simulink model "Model1_Test_Forall"  (R2018b)
settings: Solver=ode8  StartTime=0.0  StopTime=100.0  FixedStep=0.01  RelTol=1e-6
undefined symbols (not defined in the file or in its folder): tollerableriskTest_Forall
settings Model: SimulationMode=accelerator  Creator=claudio.menghi  LastModifiedBy=claudio.menghi
settings SolverCC: MaxConsecutiveZCs=10000  ShapePreserveControl=EnableAll  ZeroCrossControl=EnableAll  ZeroCrossAlgorithm=Adaptive  AutoInsertRateTranBlk=on

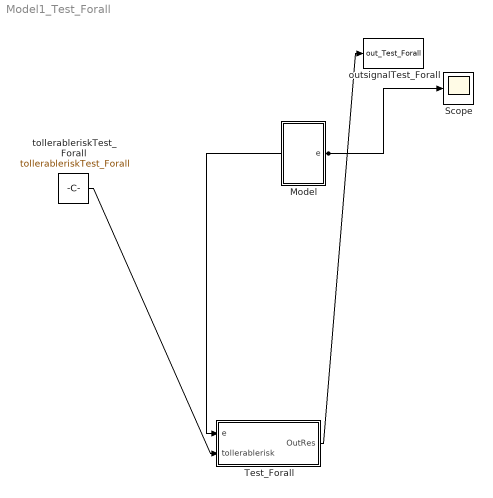
== system Model1_Test_Forall ==
  Model : Subsystem
  Scope : Scope
  Test_Forall : Subsystem
  outsignalTest_Forall : ToWorkspace  VariableName=out_Test_Forall  SaveFormat=Timeseries  SampleTime=-1
      settings: MaxDataPoints=1
  tollerableriskTest_Forall : Constant  Value=tollerableriskTest_Forall
  wires:
  Model/1(e) -> Scope/1, Test_Forall/1(e)
  tollerableriskTest_Forall/1 -> Test_Forall/2(tollerablerisk)
  Test_Forall/1(OutRes) -> outsignalTest_Forall/1

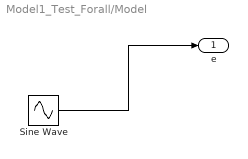
== system Model1_Test_Forall/Model ==
  Sine Wave : Sin  Amplitude=2  SampleTime=0
  e : Outport
  wires:
  Sine Wave/1 -> e/1

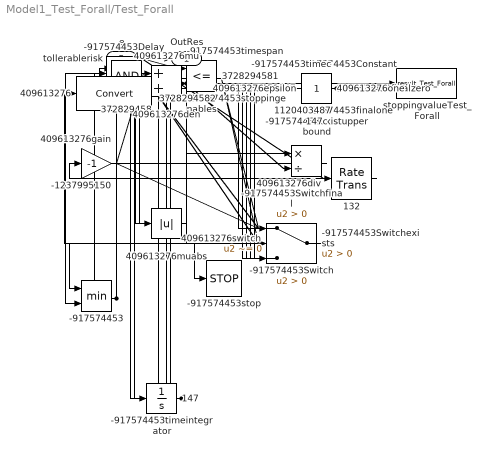
== system Model1_Test_Forall/Test_Forall ==
  e : Inport
  tollerablerisk : Inport  Port=2
  -1237995150 : Gain
  -917574453 : MinMax  Inputs=2
  -917574453Constant : Constant
  -917574453Delay : UnitDelay  InitialCondition=1  SampleTime=-1
  -917574453Switch : Switch  Criteria=u2 > Threshold
  -917574453Switchexists : Switch  Criteria=u2 > Threshold
  -917574453Switchfinal : Switch  Criteria=u2 > Threshold
  -917574453existupperbound : Constant  Value=0.0
  -917574453finalone : Constant
  -917574453finalzero : Constant  Value=0
  -917574453stop : Stop
  -917574453stoppingenables : RelationalOperator  OutDataTypeStr=boolean  RndMeth=Simplest
  -917574453timec : Constant
  -917574453timeintegrator : Integrator
  -917574453timespan : RelationalOperator  OutDataTypeStr=boolean  RndMeth=Simplest
  1065353247 : Constant  Value=1.0
  1120403487 : Constant  Value=100.0
  132 : RateTransition
  147 : Integrator
  147c : Constant
  31 : Constant  Value=0.0
  372829458 : Logic  AllPortsSameDT=off  OutDataTypeStr=boolean
  3728294581 : RelationalOperator  Operator=<=  OutDataTypeStr=boolean  RndMeth=Simplest
  3728294582 : RelationalOperator  Operator=<=  OutDataTypeStr=boolean  RndMeth=Simplest
  409613276 : DataTypeConversion
  409613276den : Sum
  409613276div : Product  Inputs=*/
  409613276epsilon : Constant  Value=-0.01
  409613276gain : Gain  Gain=-1
  409613276mu : Sum  Inputs=+-
  409613276muabs : Abs
  409613276one : Constant
  409613276switch : Switch  Criteria=u2 ~= 0
  stoppingvalueTest_Forall : ToWorkspace  VariableName=result_Test_Forall  SaveFormat=Timeseries  SampleTime=-1
      settings: MaxDataPoints=1
  OutRes : Outport
  wires:
  147c/1 -> 147/1
  31/1 -> 3728294581/1
  147/1 -> 3728294581/2, 3728294582/1
  1120403487/1 -> 3728294582/2
  3728294581/1 -> 372829458/1
  3728294582/1 -> 372829458/2
  e/1 -> 132/1
  132/1 -> -1237995150/1
  -1237995150/1 -> 409613276mu/1
  1065353247/1 -> 409613276mu/2
  409613276mu/1 -> 409613276muabs/1, 409613276div/1, 409613276switch/2
  409613276muabs/1 -> 409613276den/1
  409613276one/1 -> 409613276den/2
  409613276den/1 -> 409613276div/2
  409613276div/1 -> 409613276gain/1
  409613276gain/1 -> 409613276switch/1
  409613276epsilon/1 -> 409613276switch/3
  409613276switch/1 -> 409613276/1
  -917574453Constant/1 -> -917574453Switch/3
  372829458/1 -> -917574453Switch/2
  409613276/1 -> -917574453Switch/1
  -917574453Switch/1 -> -917574453/1
  -917574453/1 -> -917574453Delay/1, OutRes/1, -917574453timespan/2, stoppingvalueTest_Forall/1
  -917574453Delay/1 -> -917574453/2
  tollerablerisk/1 -> -917574453timespan/1
  -917574453finalzero/1 -> -917574453Switchfinal/3, -917574453Switchexists/3
  -917574453timec/1 -> -917574453timeintegrator/1
  -917574453timeintegrator/1 -> -917574453stoppingenables/1
  -917574453existupperbound/1 -> -917574453stoppingenables/2
  -917574453stoppingenables/1 -> -917574453Switchexists/2
  -917574453timespan/1 -> -917574453Switchexists/1
  -917574453finalone/1 -> -917574453Switchfinal/1
  -917574453Switchexists/1 -> -917574453Switchfinal/2
  -917574453Switchfinal/1 -> -917574453stop/1
